simulink model "ITACG"  (R2023b)
settings: Solver=ode4  StartTime=0.0  StopTime=60  FixedStep=1/100  RelTol=1e-3
libraries: simulink_extras x13, simulink x1
settings Model: NumberOfSteps=10  PacingRate=5  Creator=Administrator  LastModifiedBy=Administrator
settings DebuggingCC: UnderSpecifiedDimensionMsg=warning

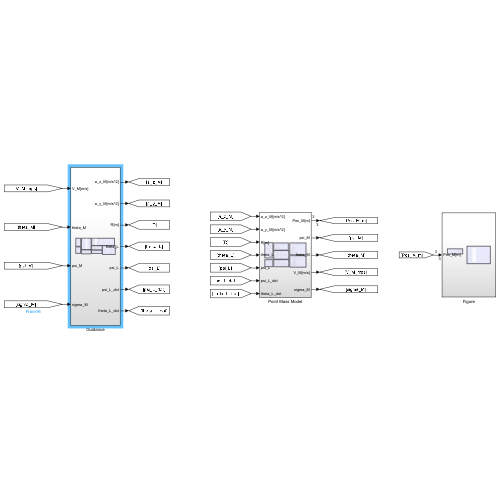
[thumbnail: Simulink's stored preview of the top-level diagram]
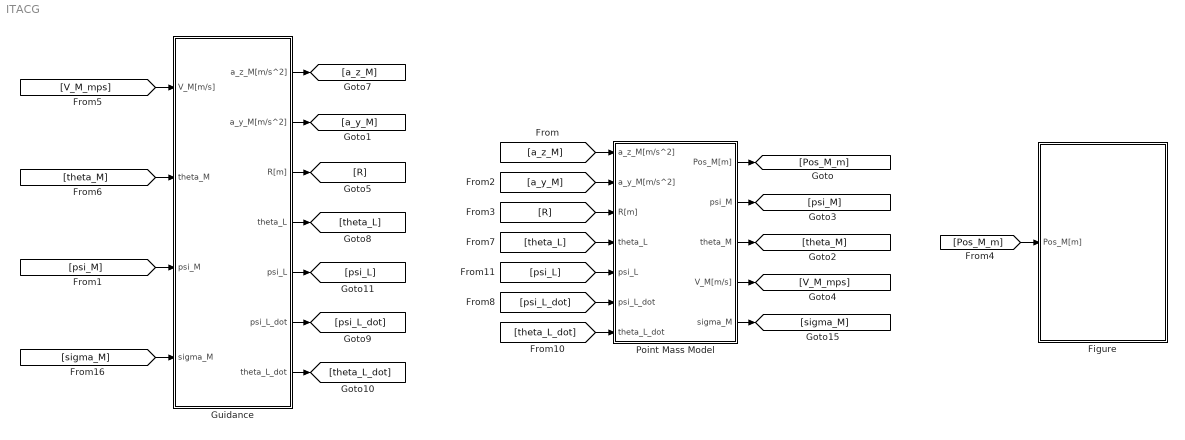
== system ITACG ==
  Figure : Subsystem
  Guidance : Subsystem
  Point Mass Model : Subsystem
  wires:
  [V_M_mps] -> Guidance/1(V_M[m/s])
  [Pos_M_m] -> Figure/1(Pos_M[m])
  [theta_M] -> Guidance/2(theta_M)
  [psi_M] -> Guidance/3(psi_M)
  Guidance/5(psi_L) -> [psi_L]
  Guidance/1(a_z_M[m/s^2]) -> [a_z_M]
  Guidance/2(a_y_M[m/s^2]) -> [a_y_M]
  Guidance/3(R[m]) -> [R]
  Guidance/4(theta_L) -> [theta_L]
  [a_z_M] -> Point Mass Model/1(a_z_M[m/s^2])
  [a_y_M] -> Point Mass Model/2(a_y_M[m/s^2])
  [R] -> Point Mass Model/3(R[m])
  [theta_L] -> Point Mass Model/4(theta_L)
  [psi_L] -> Point Mass Model/5(psi_L)
  Point Mass Model/1(Pos_M[m]) -> [Pos_M_m]
  Point Mass Model/4(V_M[m/s]) -> [V_M_mps]
  Guidance/6(psi_L_dot) -> [psi_L_dot]
  Guidance/7(theta_L_dot) -> [theta_L_dot]
  [psi_L_dot] -> Point Mass Model/6(psi_L_dot)
  [theta_L_dot] -> Point Mass Model/7(theta_L_dot)
  Point Mass Model/5(sigma_M) -> [sigma_M]
  [sigma_M] -> Guidance/4(sigma_M)
  Point Mass Model/2(psi_M) -> [psi_M]
  Point Mass Model/3(theta_M) -> [theta_M]

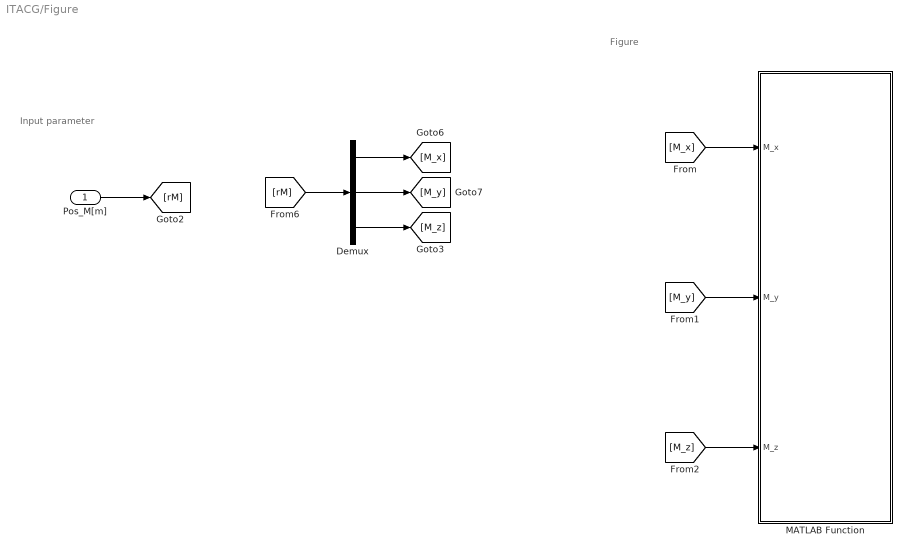
== system ITACG/Figure ==
  note: Figure
  note: Input parameter
  Pos_M[m] : Inport
  Demux : Demux  Outputs=3
  MATLAB Function : MATLAB Function  TreatAsAtomicUnit=on
  wires:
  Pos_M[m]/1 -> [rM]
  Demux/2 -> [M_y]
  Demux/1 -> [M_x]
  Demux/3 -> [M_z]
  [M_x] -> MATLAB Function/1(M_x)
  [M_y] -> MATLAB Function/2(M_y)
  [M_z] -> MATLAB Function/3(M_z)
  [rM] -> Demux/1

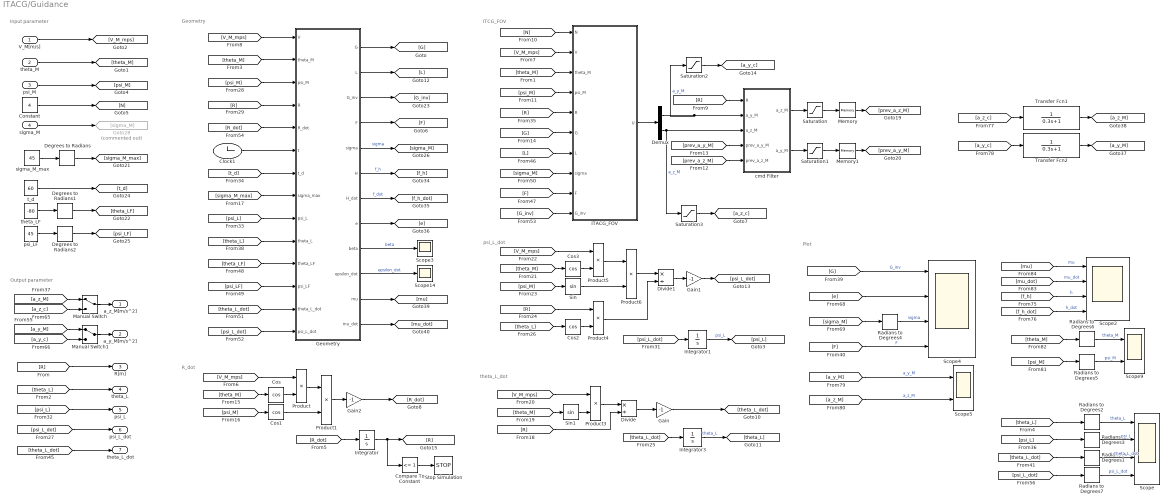
== system ITACG/Guidance ==
  note: Plot
  note: Input parameter
  note: ITCG_FOV
  note: R_dot
  note: psi_L_dot
  note: theta_L_dot
  note: Geometry
  note: Output parameter
  V_M[m/s] : Inport
  theta_M : Inport  Port=2
  psi_M : Inport  Port=3
  sigma_M : Inport  Port=4
  Clock1 : Clock
  Compare To Constant : simulink/Logic and Bit Operations/Compare To Constant  relop=<=  const=1  OutDataTypeStr=boolean
  Constant : Constant  Value=4
  Cos{,1..3} (4 alike) : Trigonometry  Operator=cos
  Degrees to Radians : simulink_extras/Transformations/Degrees to Radians
  Degrees to Radians1 : simulink_extras/Transformations/Degrees to Radians
  Degrees to Radians2 : simulink_extras/Transformations/Degrees to Radians
  Demux : Demux  Outputs=2
  Divide : Product  Inputs=*/
  Divide1 : Product  Inputs=*/
  Gain : Gain  Gain=-1
  Gain1 : Gain  Gain=-1
  Gain2 : Gain  Gain=-1
  Geometry : MATLAB Function  TreatAsAtomicUnit=on
  Goto28 : Goto  Commented=on  GotoTag=sigma_M
  ITACG_FOV : MATLAB Function  TreatAsAtomicUnit=on
  Integrator : Integrator  InitialCondition=15000
  Integrator1 : Integrator  InitialCondition=45*pi/180
  Integrator3 : Integrator  InitialCondition=-15*pi/180
  Manual Switch : ManualSwitch
  Manual Switch1 : ManualSwitch
  Memory : Memory
  Memory1 : Memory
  Product{,1,3..6} (6 alike) : Product
  Radians to Degrees{1..7} (7 alike) : simulink_extras/Transformations/Radians to Degrees
  Saturation{,1..3} (4 alike) : Saturate  UpperLimit=100  LowerLimit=-100
  Scope : Scope  NumInputPorts=4
  Scope14 : Scope
  Scope2 : Scope  NumInputPorts=4
  Scope3 : Scope
  Scope4 : Scope  NumInputPorts=4
  Scope5 : Scope  NumInputPorts=2
  Scope9 : Scope  NumInputPorts=2
  Sin : Trigonometry
  Sin1 : Trigonometry
  Stop Simulation : Stop
  Transfer Fcn1 : TransferFcn  Denominator=[0.3 1]  ParameterTunability=Optimized
  Transfer Fcn2 : TransferFcn  Denominator=[0.3 1]  ParameterTunability=Optimized
  cmd Filter : MATLAB Function  TreatAsAtomicUnit=on
  psi_LF : Constant  Value=45
  sigma_M_max : Constant  Value=45
  t_d : Constant  Value=60
  theta_LF : Constant  Value=-80
  a_z_M[m/s^2] : Outport
  a_y_M[m/s^2] : Outport  Port=2
  R[m] : Outport  Port=3
  theta_L : Outport  Port=4
  psi_L : Outport  Port=5
  psi_L_dot : Outport  Port=6
  theta_L_dot : Outport  Port=7
  wires:
  V_M[m/s]/1 -> [V_M_mps]
  Constant/1 -> [N]
  theta_M/1 -> [theta_M]
  psi_M/1 -> [psi_M]
  Product1/1 -> Gain2/1
  [R] -> Geometry/4(R)
  Gain2/1 -> [R_dot]
  [theta_L] -> Cos2/1
  [theta_L_dot] -> Integrator3/1
  [theta_M] -> Geometry/2(theta_M)
  Gain/1 -> [theta_L_dot]
  Product5/1 -> Product6/1
  Divide1/1 -> Gain1/1
  [V_M_mps] -> Product3/1
  [V_M_mps] -> Geometry/1(V)
  [psi_M] -> Geometry/3(psi_M)
  [V_M_mps] -> Product5/1
  [theta_M] -> Sin1/1
  [R] -> Divide/2
  [theta_M] -> Cos3/1
  [psi_M] -> ITACG_FOV/4(psi_M)
  Divide/1 -> Gain/1
  [theta_M] -> Cos/1
  [R] -> Product4/1
  Product4/1 -> Divide1/2
  Integrator3/1 -> [theta_L]  "theta_L"
  [psi_L_dot] -> Integrator1/1
  Sin1/1 -> Product3/2
  Product3/1 -> Divide/1
  [psi_M] -> Cos1/1
  Cos/1 -> Product/2
  Integrator1/1 -> [psi_L]  "psi_L"
  [N] -> ITACG_FOV/1(N)
  [theta_M] -> ITACG_FOV/3(theta_M)
  Product6/1 -> Divide1/1
  [psi_M] -> Sin/1
  Compare To Constant/1 -> Stop Simulation/1
  [V_M_mps] -> Product/1
  Cos3/1 -> Product5/2
  Sin/1 -> Product6/2
  Integrator/1 -> [R], Compare To Constant/1
  [R] -> ITACG_FOV/5(R)
  Product/1 -> Product1/1
  Cos2/1 -> Product4/2
  Cos1/1 -> Product1/2
  Gain1/1 -> [psi_L_dot]
  [R_dot] -> Integrator/1
  [V_M_mps] -> ITACG_FOV/2(V)
  [theta_L] -> theta_L/1
  [psi_L] -> psi_L/1
  [R] -> R[m]/1
  Clock1/1 -> Geometry/6(t)
  sigma_M_max/1 -> Degrees to Radians/1
  Degrees to Radians/1 -> [sigma_M_max]
  [sigma_M_max] -> Geometry/8(sigma_max)
  t_d/1 -> [t_d]
  [t_d] -> Geometry/7(t_d)
  [R] -> cmd Filter/1(R)
  Memory/1 -> [prev_a_z_M]
  Memory1/1 -> [prev_a_y_M]
  [prev_a_z_M] -> cmd Filter/5(prev_a_z_M)
  [prev_a_y_M] -> cmd Filter/4(prev_a_y_M)
  [psi_L_dot] -> psi_L_dot/1
  [theta_L_dot] -> theta_L_dot/1
  ITACG_FOV/1(U) -> Demux/1
  Geometry/1(G) -> [G]
  Geometry/2(L) -> [L]
  [G] -> ITACG_FOV/6(G)
  [L] -> ITACG_FOV/7(L)
  [psi_L] -> Geometry/9(psi_L)
  [theta_L] -> Geometry/10(theta_L)
  theta_LF/1 -> Degrees to Radians1/1
  psi_LF/1 -> Degrees to Radians2/1
  [theta_LF] -> Geometry/11(theta_LF)
  [psi_LF] -> Geometry/12(psi_LF)
  [sigma_M] -> ITACG_FOV/8(sigma)
  [theta_L_dot] -> Geometry/13(theta_L_dot)
  [psi_L_dot] -> Geometry/14(psi_L_dot)
  Degrees to Radians1/1 -> [theta_LF]
  Degrees to Radians2/1 -> [psi_LF]
  Geometry/3(G_inv) -> [G_inv]
  Geometry/4(F) -> [F]
  [F] -> ITACG_FOV/9(F)
  [R_dot] -> Geometry/5(R_dot)
  cmd Filter/1(a_z_M) -> Saturation/1
  cmd Filter/2(a_y_M) -> Saturation1/1
  sigma_M/1 -> Goto28/1
  Geometry/5(sigma) -> [sigma_M]  "sigma"
  Demux/1 -> Saturation2/1, cmd Filter/2("a_y_M ")  "a_y_M"
  Demux/2 -> cmd Filter/3("a_z_M "), Saturation3/1  "a_z_M"
  [a_z_M] -> Manual Switch/1
  [a_z_c] -> Manual Switch/2
  Manual Switch/1 -> a_z_M[m/s^2]/1
  [a_y_M] -> Manual Switch1/1
  [a_y_c] -> Manual Switch1/2
  Manual Switch1/1 -> a_y_M[m/s^2]/1
  Geometry/6(H) -> [f_h]  "f_h"
  Geometry/7(H_dot) -> [f_h_dot]  "f_dot"
  [G_inv] -> ITACG_FOV/10(G_inv)
  [e] -> Scope4/2
  [sigma_M] -> Radians to Degrees4/1
  [F] -> Scope4/4  "F"
  Radians to Degrees4/1 -> Scope4/3  "sigma"
  [G] -> Scope4/1  "G_inv"
  [f_h] -> Scope2/3  "h"
  [f_h_dot] -> Scope2/4  "h_dot"
  Geometry/9(beta) -> Scope3/1  "beta"
  [a_z_M] -> Scope5/2  "a_z_M"
  [a_y_M] -> Scope5/1  "a_y_M"
  Saturation/1 -> Memory/1
  Saturation1/1 -> Memory1/1
  Geometry/10(epsilon_dot) -> Scope14/1  "epsilon_dot"
  [theta_M] -> Radians to Degrees6/1
  [psi_M] -> Radians to Degrees5/1
  Radians to Degrees5/1 -> Scope9/2  "psi_M"
  Radians to Degrees6/1 -> Scope9/1  "theta_M"
  Geometry/11(mu) -> [mu]
  Geometry/12(mu_dot) -> [mu_dot]
  [mu] -> Scope2/1  "mu"
  [mu_dot] -> Scope2/2  "mu_dot"
  Geometry/8(e) -> [e]
  [theta_L] -> Radians to Degrees2/1
  [psi_L] -> Radians to Degrees3/1
  [a_z_c] -> Transfer Fcn1/1
  Transfer Fcn1/1 -> [a_z_M]
  [a_y_c] -> Transfer Fcn2/1
  Transfer Fcn2/1 -> [a_y_M]
  [theta_L_dot] -> Radians to Degrees1/1
  [psi_L_dot] -> Radians to Degrees7/1
  Radians to Degrees2/1 -> Scope/1  "theta_L"
  Radians to Degrees3/1 -> Scope/2  "psi_L"
  Radians to Degrees1/1 -> Scope/3  "theta_L_dot"
  Radians to Degrees7/1 -> Scope/4  "psi_L_dot"
  Saturation2/1 -> [a_y_c]
  Saturation3/1 -> [a_z_c]

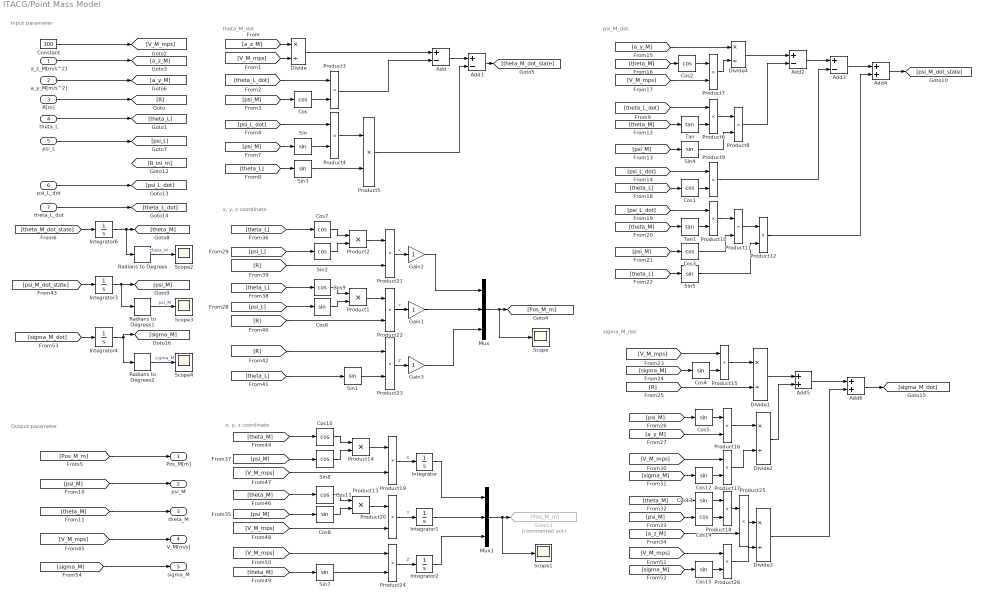
== system ITACG/Point Mass Model ==
  note: sigma_M_dot
  note: Input parameter
  note: x, y, z coordinate
  note: theta_M_dot
  note: Output parameter
  note: psi_M_dot
  note: x, y, z coordinate
  a_z_M[m/s^2] : Inport
  a_y_M[m/s^2] : Inport  Port=2
  R[m] : Inport  Port=3
  theta_L : Inport  Port=4
  psi_L : Inport  Port=5
  psi_L_dot : Inport  Port=6
  theta_L_dot : Inport  Port=7
  Add{,1..3} (4 alike) : Sum  Inputs=+-
  Add4 : Sum
  Add5 : Sum
  Add6 : Sum
  Constant : Constant  Value=300
  Cos{,1..3,7,9..11,14} (9 alike) : Trigonometry  Operator=cos
  Cos{4..6,8,12..13,15} (7 alike) : Trigonometry
  Divide{,1..4} (5 alike) : Product  Inputs=*/
  Gain1 : Gain
  Gain2 : Gain
  Gain3 : Gain
  Goto11 : Goto  Commented=on  GotoTag=Pos_M_m
  Integrator : Integrator
  Integrator1 : Integrator
  Integrator2 : Integrator
  Integrator3 : Integrator  InitialCondition=0*pi/180
  Integrator4 : Integrator  InitialCondition=10*pi/180
  Integrator6 : Integrator  InitialCondition=10*pi/180
  Mux : Mux  Inputs=3
  Mux1 : Mux  Inputs=3
  Product{1..26} (26 alike) : Product
  Radians to Degrees : simulink_extras/Transformations/Radians to Degrees
  Radians to Degrees1 : simulink_extras/Transformations/Radians to Degrees
  Radians to Degrees2 : simulink_extras/Transformations/Radians to Degrees
  Scope{,1..4} (5 alike) : Scope
  Sin{,1,3..5,7} (6 alike) : Trigonometry
  Sin2 : Trigonometry  Operator=cos
  Sin8 : Trigonometry  Operator=cos
  Tan : Trigonometry  Operator=tan
  Tan1 : Trigonometry  Operator=tan
  Pos_M[m] : Outport
  psi_M : Outport  Port=2
  theta_M : Outport  Port=3
  V_M[m/s] : Outport  Port=4
  sigma_M : Outport  Port=5
  wires:
  [psi_M] -> psi_M/1
  [theta_L] -> Cos9/1
  [V_M_mps] -> Divide/2
  [V_M_mps] -> V_M[m/s]/1
  Add2/1 -> Add3/1
  Add1/1 -> [theta_M_dot_state]
  [a_z_M] -> Divide/1
  Add3/1 -> Add4/1
  [a_y_M] -> Divide4/1
  Divide4/1 -> Add2/1
  theta_L/1 -> [theta_L]
  [V_M_mps] -> Product7/2
  Cos6/1 -> Product1/2
  a_y_M[m/s^2]/1 -> [a_y_M]
  Product23/1 -> Gain3/1  "Z"
  [Pos_M_m] -> Pos_M[m]/1
  Integrator6/1 -> Radians to Degrees/1, [theta_M]
  [psi_L] -> Cos6/1
  Add/1 -> Add1/1
  psi_L/1 -> [psi_L]
  Product21/1 -> Gain2/1  "X"
  Product1/1 -> Product22/1
  Integrator3/1 -> Radians to Degrees1/1, [psi_M]
  Sin2/1 -> Product2/2
  a_z_M[m/s^2]/1 -> [a_z_M]
  Add4/1 -> [psi_M_dot_state]
  Cos2/1 -> Product7/1
  Mux/1 -> [Pos_M_m], Scope/1
  R[m]/1 -> [R]
  [theta_M] -> theta_M/1
  [psi_L] -> Sin2/1
  [theta_M] -> Cos2/1
  Product2/1 -> Product21/1
  Cos9/1 -> Product1/1
  [theta_L] -> Cos7/1
  Product7/1 -> Divide4/2
  Divide/1 -> Add/1
  Cos7/1 -> Product2/1
  Product22/1 -> Gain1/1  "Y"
  [V_M_mps] -> Product24/1
  Sin7/1 -> Product24/2
  [V_M_mps] -> Product20/2
  [theta_M] -> Cos11/1
  [psi_M] -> Sin8/1
  Mux1/1 -> Scope1/1, Goto11/1
  [theta_M] -> Sin7/1
  Sin8/1 -> Product14/2
  Product14/1 -> Product19/1
  Product19/1 -> Integrator/1  "X"
  Product13/1 -> Product20/1
  Product24/1 -> Integrator2/1  "Z"
  [psi_M] -> Cos8/1
  [V_M_mps] -> Product19/2
  [theta_M] -> Cos10/1
  Cos11/1 -> Product13/1
  Cos8/1 -> Product13/2
  Product20/1 -> Integrator1/1  "Y"
  Cos10/1 -> Product14/1
  Integrator/1 -> Mux1/1
  Integrator1/1 -> Mux1/2
  ? -> [R_ini_m]
  [R] -> Product21/2
  [R] -> Product22/2
  Gain1/1 -> Mux/2
  Gain2/1 -> Mux/1
  [R] -> Product23/1
  Sin1/1 -> Product23/2
  [theta_L] -> Sin1/1
  [theta_L_dot] -> Product3/1
  [psi_M] -> Cos/1
  Cos/1 -> Product3/2
  Product3/1 -> Add/2
  [psi_M] -> Sin/1
  [psi_L_dot] -> Product4/1
  Sin/1 -> Product4/2
  Product4/1 -> Product5/1
  [theta_L] -> Sin3/1
  Sin3/1 -> Product5/2
  Product5/1 -> Add1/2
  psi_L_dot/1 -> [psi_L_dot]
  theta_L_dot/1 -> [theta_L_dot]
  [theta_L_dot] -> Product6/1
  [theta_M] -> Tan/1
  Tan/1 -> Product6/2
  [psi_M] -> Sin4/1
  Product6/1 -> Product8/1
  Sin4/1 -> Product8/2
  Product8/1 -> Add2/2
  [psi_L_dot] -> Product9/1
  Cos1/1 -> Product9/2
  [theta_L] -> Cos1/1
  Product9/1 -> Add3/2
  [theta_M] -> Tan1/1
  Tan1/1 -> Product10/2
  [psi_L_dot] -> Product10/1
  Product10/1 -> Product11/1
  [psi_M] -> Cos3/1
  Cos3/1 -> Product11/2
  [theta_L] -> Sin5/1
  Product11/1 -> Product12/1
  Sin5/1 -> Product12/2
  Product12/1 -> Add4/2
  Radians to Degrees/1 -> Scope2/1  "theta_M"
  Radians to Degrees1/1 -> Scope3/1  "psi_M"
  [V_M_mps] -> Product15/1
  Cos4/1 -> Product15/2
  [sigma_M] -> Cos4/1
  Product15/1 -> Divide1/1
  [R] -> Divide1/2
  Divide1/1 -> Add5/1
  [psi_M] -> Cos5/1
  Cos5/1 -> Product16/1
  [a_y_M] -> Product16/2
  Product16/1 -> Divide2/1
  [V_M_mps] -> Product17/1
  [sigma_M] -> Cos12/1
  Cos12/1 -> Product17/2
  Product17/1 -> Divide2/2
  Divide2/1 -> Add5/2
  Add5/1 -> Add6/1
  [theta_M] -> Cos13/1
  [psi_M] -> Cos14/1
  Cos13/1 -> Product18/1
  Cos14/1 -> Product18/2
  Product18/1 -> Product25/1
  [a_z_M] -> Product25/2
  Product25/1 -> Divide3/1
  Cos15/1 -> Product26/2
  [V_M_mps] -> Product26/1
  [sigma_M] -> Cos15/1
  Product26/1 -> Divide3/2
  Divide3/1 -> Add6/2
  Add6/1 -> [sigma_M_dot]
  [sigma_M_dot] -> Integrator4/1
  Integrator4/1 -> [sigma_M], Radians to Degrees2/1
  Radians to Degrees2/1 -> Scope4/1  "sigma_M"
  [sigma_M] -> sigma_M/1
  [theta_M_dot_state] -> Integrator6/1
  [psi_M_dot_state] -> Integrator3/1
  Integrator2/1 -> Mux1/3
  Gain3/1 -> Mux/3
  Constant/1 -> [V_M_mps]

== matlab function ITACG/Guidance/ITACG_FOV ==
  data: U output; N input; V input; theta_M input; psi_M input; R input; G input; L input; sigma input; F input; G_inv input
function U   = fcn(N, V, theta_M, psi_M, R, G, L, sigma, F, G_inv)
    D2R = 180/pi;
    sigma_s = 0.001 * D2R;
    % sigma_deg = sigma*180/pi;
    U_PN = [-sin(psi_M) -sin(theta_M)*cos(psi_M)]';
    %% G_inv
    % U_eq = G_inv * F;

    % if abs(sigma) > sigma_s
    %     U = G_inv * L + U_eq;
    % else
    %     U = N * V^2 * U_PN / R;
    % end
    % U = G_inv * L + U_eq;

    %% G^-1
    U_eq = G^-1 * F;

    if abs(sigma) > sigma_s
        U = G^-1 * L - U_eq;
    else
        U = N * V^2 * U_PN / R;
    end

== matlab function ITACG/Guidance/Geometry ==
  data: V input; theta_M input; psi_M input; R input; R_dot input; t input; t_d input; sigma_max input; G output; L output; psi_L input; theta_L input; theta_LF input; psi_LF input; theta_L_dot input; psi_L_dot input; G_inv output; F output; sigma output; H output; H_dot output; e output; beta output; epsilon_dot output; mu output; mu_dot output
function [G, L, G_inv, F, sigma, H, H_dot, e, beta, epsilon_dot, mu, mu_dot] =fcn(V, theta_M, psi_M, R, R_dot, t, t_d, sigma_max, psi_L, theta_L, theta_LF, psi_LF, theta_L_dot, psi_L_dot)
    %% constant parameter
    b= 0.1;
    k= 1.4;
    eta = 0.5;
    T_s = 0.6 * t_d;

    %% guidance parameter
    sigma = acos(cos(theta_M) * cos(psi_M));
    t_go = t_d - t;

    %% epsilon
    epsilon = t_go - R / V;
    epsilon_dot = cos(sigma) - 1;

    %% theta_e
    theta_e = theta_L - theta_LF;
    theta_e_dot = theta_L_dot;

    %% psi_e
    psi_e = psi_L - psi_LF;
    psi_e_dot = psi_L_dot;

    %% beta
    beta = (theta_e^2 + cos(theta_L)^2 * psi_e^2) / (4 * V^2);
    % beta = sin(sigma)^2 * theta_e / (4 * V^2 * sin(theta_M)^2);

    beta_dot = (theta_e * theta_e_dot + cos(theta_L)^2 * psi_e * psi_e_dot - sin(theta_L) * cos(theta_L) * psi_e^2 * theta_L_dot) / (2 * V^2);

    %% C_f/C_g  
    C_f = psi_e * sin(theta_L) * cos(theta_L);
    C_g = psi_e * cos(theta_M) * cos(theta_L) + theta_e * sin(theta_M) * sin(psi_M);

    %% H
    H = (2 * epsilon^2) / (beta * R^2 + epsilon^2);
    H_dot = ((4 * epsilon * epsilon_dot) / (beta * R^2 + epsilon^2)) - ((2 * epsilon^2 * (beta_dot * R^2 + 2 * beta * R * R_dot + 2 * epsilon * epsilon_dot)) / (beta * R^2 + epsilon^2)^2);
    H_max = 1 - cos(sigma_max);
    H_bar = H / H_max;

    %% chi
    if abs(theta_L) >= pi/2
        chi = theta_e * sin(theta_M);
    else
        chi = psi_e * cos(theta_M) * cos(theta_L) * sin(psi_M) + theta_e * sin(theta_M);
    end
    %% F(H)
    if H < eta * H_max
        f_h = H;
    else
        f_h = ((1 - eta) * tanh((H_bar - eta) / (1 - eta)) + eta) * H_max;
    end
    %% F(H)_dot
    if H < eta * H_max
        f_h_dot = H_dot;
    else
        f_h_dot = (1 - tanh((H_bar - eta) / (1 - eta))^2) * H_dot;
    end

    %% mu    
    if t >= 0 && t < T_s
        mu = T_s / (T_s - t);
        mu_dot = T_s / (T_s - t)^2;
    else
        mu = 1;
        mu_dot = 0;
    end

    %% Baseline Error Dynamics
    % e = [epsilon_dot + H;
    %     psi_e * theta_e_dot - theta_e * psi_e_dot];
    % 
    % F = [-R * theta_L_dot^2 / V - R * psi_L_dot^2 * cos(theta_L)^2 / V + H_dot;
    %     2 * (theta_e * psi_L_dot - psi_e * theta_L_dot) * R_dot / R - C_f * psi_L_dot^2 - 2 * theta_e * psi_L_dot * theta_L_dot * tan(theta_L)]; 

    %% Nonlinear Error Dynamics
    e = [epsilon_dot + f_h;
        psi_e * theta_e_dot - theta_e * psi_e_dot];

    F = [-R * theta_L_dot^2 / V - R * psi_L_dot^2 * cos(theta_L)^2 / V + f_h_dot;
        2 * (theta_e * psi_L_dot - psi_e * theta_L_dot) * R_dot / R - C_f * psi_L_dot^2 - 2 * theta_e * psi_L_dot * theta_L_dot * tan(theta_L)]; 

    %% guidance vector
    G = [-sin(psi_M) / V, -sin(theta_M) * cos(psi_M) / V;
        theta_e * cos(psi_M) / (R * cos(theta_L)), -C_g / (R * cos(theta_L))];

    G_inv = 1 / chi * [-V * C_g, R * sin(theta_M) * cos(psi_M) * cos(theta_L);
        -V * theta_e * cos(psi_M), -R * sin(psi_M) * cos(theta_L)];

    % ne = norm(e);
    L = -(b + k * mu_dot / mu) * e;

== matlab function ITACG/Figure/MATLAB Function ==
  settings: updateMethod=DISCRETE
  data: M_x input; M_y input; M_z input
function fcn(M_x, M_y, M_z)

persistent data timeldx
if isempty(data)      
    data=zeros(100000,3);
    timeldx=1;
end


pos_missile=zeros(1,3);
pos_missile(1,2)=M_x;
pos_missile(1,1)=M_y;
pos_missile(1,3)=-M_z;



data(timeldx,:)=pos_missile;

plot3(data(1:timeldx,2), data(1:timeldx,1), data(1:timeldx, 3));
grid;
hold on;
plot3(0,0, 00, '*');

plot3(M_x, M_y, -M_z, 'rpentagram', 'LineWidth',1);

plot3(data(1:timeldx,2), data(1:timeldx,1), data(1:timeldx,3));


title('Impact Time Angle Control Guidance')
xlabel('X(m)')
ylabel('Y(m)')
zlabel('Z(m)')
hold off;
% xlim([000 11000]);
% ylim([0 11000]);
% zlim([0 6000]);
timeldx=timeldx+1;

end

== matlab function ITACG/Guidance/cmd Filter ==
  data: R input; a_y_M input; a_z_M output; a_z_M input; prev_a_y_M input; prev_a_z_M input; a_y_M output
function [a_z_M, a_y_M] = fcn(R, a_y_M, a_z_M, prev_a_y_M, prev_a_z_M)

if R<10
    a_z_M = prev_a_z_M;
    a_y_M = prev_a_y_M;
end
